simulink model "servoStateControl"  (R2024b)
settings: Solver=VariableStepAuto  StartTime=0.0  StopTime=1  RelTol=1e-3
undefined symbols (not defined in the file): A, B, C, K, x_0, x_s
settings Model: Creator=Longbin  LastModifiedBy=Longbin

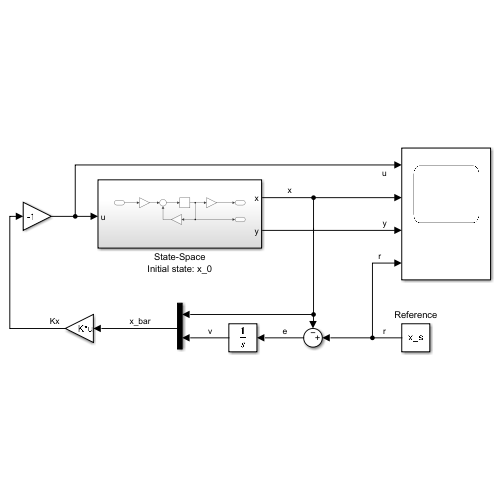
[thumbnail: Simulink's stored preview of the top-level diagram]
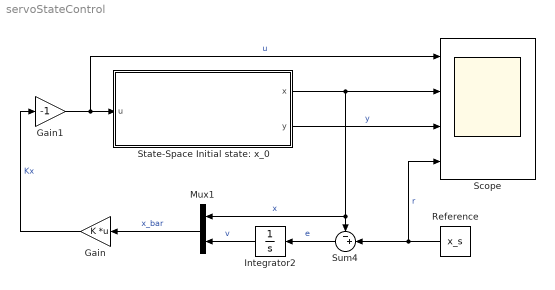
== system servoStateControl ==
  Gain : Gain  Gain=K  Multiplication=Matrix(K*u)
  Gain1 : Gain  Gain=-1
  Integrator2 : Integrator
  Mux1 : Mux  Inputs=2
  Reference : Constant  Value=x_s
  Scope : Scope  NumInputPorts=4
  State-Space Initial state: x_0 : Subsystem
  Sum4 : Sum  Inputs=-+|
  wires:
  Gain/1 -> Gain1/1  "Kx"
  Gain1/1 -> State-Space Initial state: x_0/1(u), Scope/1  "u"
  Integrator2/1 -> Mux1/2  "v"
  Sum4/1 -> Integrator2/1  "e"
  Reference/1 -> Scope/4, Sum4/2  "r"
  Mux1/1 -> Gain/1  "x_bar"
  State-Space Initial state: x_0/2(y) -> Scope/3  "y"
  State-Space Initial state: x_0/1(x) -> Mux1/1, Sum4/1, Scope/2  "x"

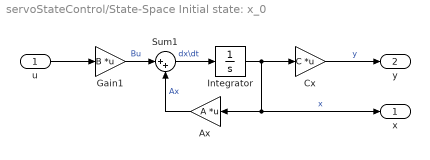
== system servoStateControl/State-Space Initial state: x_0 ==
  u : Inport
  Ax : Gain  Gain=A  Multiplication=Matrix(K*u)
  Cx : Gain  Gain=C  Multiplication=Matrix(K*u)
  Gain1 : Gain  Gain=B  Multiplication=Matrix(K*u)
  Integrator : Integrator  InitialCondition=x_0
  Sum1 : Sum  Inputs=|++
  x : Outport
  y : Outport  Port=2
  wires:
  Gain1/1 -> Sum1/1  "Bu"
  u/1 -> Gain1/1
  Ax/1 -> Sum1/2  "Ax"
  Sum1/1 -> Integrator/1  "dx\\dt"
  Integrator/1 -> Cx/1, x/1, Ax/1  "x"
  Cx/1 -> y/1  "y"
